simulink model "simulink_30_03"  (R2021a)
settings: Solver=FixedStepAuto  StartTime=0.0  StopTime=200  FixedStep=0.02  RelTol=1e-6
undefined symbols (not defined in the file): D_e, J_c, psi_sig, U_sig, V_sig
libraries: pid_lib x6, simulink x5, sharedutil x5, dspswit3 x1, aerolibutil x1
(part 1 of 3)
settings Model: Creator=frede  LastModifiedBy=frede
settings DataIOCC: SaveFormat=StructureWithTime  ReturnWorkspaceOutputs=off
settings OptimizationCC: BlockReduction=off  BufferReuse=off
settings DebuggingCC: AlgebraicLoopMsg=none  UnconnectedInputMsg=none  UnconnectedOutputMsg=none  UnconnectedLineMsg=none

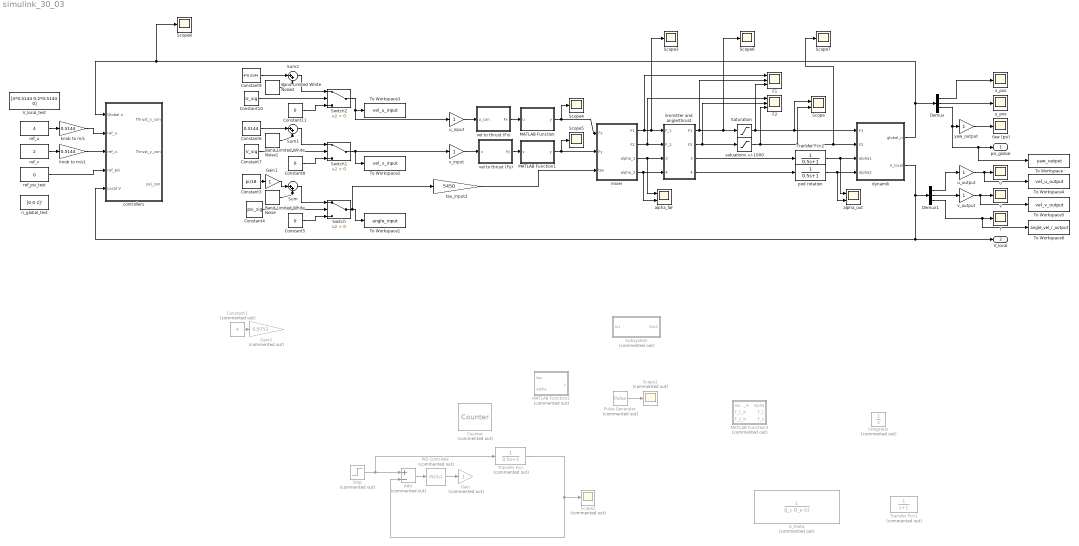
== system simulink_30_03 ==
  Add : Sum  Commented=on  Inputs=+-
  Band-Limited White Noise : simulink/Sources/Band-Limited White Noise  Cov=[0.01]  Ts=0.1  seed=[23341]
  Band-Limited White Noise1 : simulink/Sources/Band-Limited White Noise  Cov=[0.01]  Ts=0.1  seed=[23341]
  Band-Limited White Noise2 : simulink/Sources/Band-Limited White Noise  Cov=[0.01]  Ts=0.1  seed=[23341]
  Constant1 : Constant  Commented=on  Value=4
  Constant10 : Constant  Value=U_sig
  Constant11 : Constant  Value=0
  Constant3 : Constant  Value=pi/18
  Constant4 : Constant  Value=psi_sig
  Constant5 : Constant  Value=0
  Constant6 : Constant  Value=0.5144
  Constant7 : Constant  Value=V_sig
  Constant8 : Constant  Value=0
  Constant9 : Constant  Value=4*0.5144
  Counter : dspswit3/Counter  Commented=on  Direction=Up  CountEvent=Rising edge  CounterSize=User defined  MaxCount=500  InitialCount=0  Output=Count and Hit  HitValue=32  ResetInput=on  SamplesPerFrame=1  Ts=1  CntDtype=double  HitDtype=Logical
  Demux : Demux  Outputs=3
  Demux1 : Demux  Outputs=3
  F1 : Scope  NumInputPorts=3
  F2 : Scope  NumInputPorts=3
  G_theta : TransferFcn  Commented=on  Denominator=[J_c D_e 0]
  Gain : Gain  Commented=on
  Gain1 : Gain
  Gain3 : Gain  Commented=on  Gain=0.9752
  Integrator : Integrator  Commented=on
  MATLAB Function : MATLAB Function  TreatAsAtomicUnit=on
  MATLAB Function1 : MATLAB Function  TreatAsAtomicUnit=on
  MATLAB Function2 : MATLAB Function  Commented=on  TreatAsAtomicUnit=on
  MATLAB Function3 : MATLAB Function  Commented=on  TreatAsAtomicUnit=on
  PID Controller : pid_lib/PID Controller  Commented=on  Controller=PID  Form=Parallel  TimeDomain=Continuous-time  UseExternalTs=off  SampleTime=-1  IntegratorMethod=Forward Euler  FilterMethod=Forward Euler  ControllerParametersSource=internal  P=1.8562414179979  I=1.03694595494162  D=-0.170611805707441  UseFilter=on  N=7.0571761358123  TunerSelectOption=Transfer Function Based (PID Tuner App)  InitialConditionSource=internal  InitialConditionForIntegrator=0  InitialConditionForFilter=0  DifferentiatorICPrevScaledInput=0  ExternalReset=none  TrackingMode=off  Kt=1  LimitOutput=off  SatLimitsSource=internal  UpperSaturationLimit=inf  LowerSaturationLimit=-inf  LinearizeAsGain=on  AntiWindupMode=none  Kb=1  POutMin=[]  POutMax=[]  IOutMin=[]  IOutMax=[]  DOutMin=[]  DOutMax=[]  NOutMin=[]  NOutMax=[]  SumOutMin=[]  SumOutMax=[]  SaturationOutMin=[]  SaturationOutMax=[]  PParamMin=[]  PParamMax=[]  IParamMin=[]  IParamMax=[]  DParamMin=[]  DParamMax=[]  NParamMin=[]  NParamMax=[]  KbParamMin=[]  KbParamMax=[]  KtParamMin=[]  KtParamMax=[]  KbOutMin=[]  KbOutMax=[]  KtOutMin=[]  KtOutMax=[]  IntegratorOutMin=[]  IntegratorOutMax=[]  FilterOutMin=[]  FilterOutMax=[]  SumI1OutMin=[]  SumI1OutMax=[]  SumI2OutMin=[]  SumI2OutMax=[]  SumI3OutMin=[]  SumI3OutMax=[]  SumI4OutMin=[]  SumI4OutMax=[]  SumDOutMin=[]  SumDOutMax=[]  DifferentiatorOutMin=[]  DifferentiatorOutMax=[]  FilterDiffOutCoefMin=[]  FilterDiffOutCoefMax=[]  ReciprocalOutMin=[]  ReciprocalOutMax=[]  SumDenOutMin=[]  SumDenOutMax=[]  SumNumOutMin=[]  SumNumOutMax=[]  DivideOutMin=[]  DivideOutMax=[]  UdiffTsProdOutMin=[]  UdiffTsProdOutMax=[]  NTsProdOutMin=[]  NTsProdOutMax=[]  UintegralTsProdOutMin=[]  UintegralTsProdOutMax=[]  UngainTsProdOutMin=[]  UngainTsProdOutMax=[]  IntegratorContinuousStateAttributes=''  IntegratorStateMustResolveToSignalObject=off  IntegratorRTWStateStorageClass=Auto  FilterContinuousStateAttributes=''  FilterStateMustResolveToSignalObject=off  FilterRTWStateStorageClass=Auto  ParallelPVariant=InternalParameters  IdealPVariant=Disabled  IVariant=InternalParameters  DVariant=InternalParameters  IntegratorVariant=Continuous  SatVariant=Disabled  AWVariant=Passthrough  PCopyVariant=Disabled  TRVariant=Disabled  FdbkBlocksVariant=Forward  IdealPFdbkVariant=Disabled  SatFdbkVariant=Disabled  DerivativeFilterVariant=ContFilter  NVariant=InternalParameters  NCopyVariant=Disabled  FilterICVariant=InternalICsFilter  IntegratorICVariant=InternalICs  ExternalResetVariant=Disabled  TRSumVariant=Passthrough  SumFdbkVariant=Disabled  SumVariant=Sum_PID  TsampFilterVariant=InternalTs  TsampNgainVariant=Passthrough  TsampIntegralVariant=Passthrough  ExternalSaturationOutDataTypeStr=Inherit: Same as second input
  Pulse Generator : DiscretePulseGenerator  Commented=on  PulseType=Time based  Period=0.02222  PulseWidth=5
  Saturation : Saturate  UpperLimit=1000  LowerLimit=-1000
  Scope : Scope  NumInputPorts=2
  Scope1 : Scope  Commented=on
  Scope2 : Scope  Commented=on
  Scope{3..8} (6 alike) : Scope
  Step : Step  Commented=on  Time=0  After=0.78  SampleTime=0
  Subsystem : Subsystem  Commented=on
  Sum : Sum  Inputs=|++
  Sum1 : Sum  Inputs=|++
  Sum2 : Sum  Inputs=|++
  Switch : Switch  Criteria=u2 > Threshold
  Switch1 : Switch  Criteria=u2 > Threshold
  Switch2 : Switch  Criteria=u2 > Threshold
  To Workspace : ToWorkspace  VariableName=yaw_output  SaveFormat=Timeseries  SampleTime=-1
  To Workspace1 : ToWorkspace  VariableName=angle_input  SaveFormat=Timeseries  SampleTime=-1
  To Workspace2 : ToWorkspace  VariableName=vel_v_input  SaveFormat=Timeseries  SampleTime=-1
  To Workspace3 : ToWorkspace  VariableName=vel_u_input  SaveFormat=Timeseries  SampleTime=-1
  To Workspace4 : ToWorkspace  VariableName=vel_u_output  SaveFormat=Timeseries  SampleTime=-1
  To Workspace5 : ToWorkspace  VariableName=vel_v_output  SaveFormat=Timeseries  SampleTime=-1
  To Workspace6 : ToWorkspace  VariableName=angle_vel_r_output  SaveFormat=Timeseries  SampleTime=-1
  Transfer Fcn : TransferFcn  Commented=on  Denominator=[0.5 1]
  Transfer Fcn1 : TransferFcn  Commented=on  Denominator=[1 1]
  Transfer Fcn2 : TransferFcn  Denominator=[0.5 1]
  V_local_test : Constant  Value=[4*0.5144 0.2*0.5144 0]
  Yaw (psi) : Scope
  alpha_før : Scope  NumInputPorts=2
  alpha_out : Scope  NumInputPorts=2
  controllers : Subsystem
  dynamik : Subsystem
  knob to m/s : Gain  Gain=0.5144
  knob to m/s1 : Gain  Gain=0.5144
  "limmitter and angle/thrust " : MATLAB Function  TreatAsAtomicUnit=on
  mixer : Subsystem
  n_global_test : Constant  Value=[0 0 2]'
  pod rotation : TransferFcn  Denominator=[0.5 1]
  r : Scope
  ref_psi_test : Constant  Value=0
  ref_u : Constant  Value=4
  ref_v : Constant  Value=2
  "satuations +/-1000 " : Saturate  UpperLimit=1000  LowerLimit=-1000
  tau_input2 : Gain  Gain=5450
  u : Scope
  u_input : Gain
  u_output : Gain
  v : Scope
  v_input : Gain
  v_output : Gain
  vel to thrust (Fx) : MATLAB Function  TreatAsAtomicUnit=on
  vel to thrust (Fy) : MATLAB Function  TreatAsAtomicUnit=on
  x_pos : Scope
  y_pos : Scope
  yaw_output : Gain
  psi_global : Outport
  V_local : Outport  Port=2
  wires:
  yaw_output/1 -> Yaw (psi)/1
  Pulse Generator/1 -> Scope1/1
  ref_v/1 -> knob to m/s1/1
  v_output/1 -> To Workspace5/1, v/1
  tau_input2/1 -> mixer/3(tau)
  Demux/2 -> y_pos/1
  ref_u/1 -> knob to m/s/1
  vel to thrust (Fy)/1(Fy) -> MATLAB Function1/1(v)
  ref_psi_test/1 -> controllers/4(ref_psi.)
  Demux1/2 -> v_output/1
  knob to m/s/1 -> controllers/2(ref_u.)
  knob to m/s1/1 -> controllers/3(ref_v.)
  Demux1/1 -> u_output/1
  Sum/1 -> Switch/1
  Demux/1 -> x_pos/1
  dynamik/2(V_local) -> controllers/5(Local V), V_local/1, Demux1/1
  Demux/3 -> yaw_output/1, To Workspace/1, psi_global/1
  dynamik/1(global_n) -> Scope8/1, controllers/1(Global n), Demux/1
  vel to thrust (Fx)/1(Fx) -> MATLAB Function/1(u)
  Add/1 -> PID Controller/1
  Step/1 -> Transfer Fcn/1, Add/1
  Transfer Fcn/1 -> Scope2/1, Add/2
  PID Controller/1 -> Gain/1
  Transfer Fcn2/1 -> alpha_out/1, dynamik/3(alpha1)
  pod rotation/1 -> alpha_out/2, dynamik/4(alpha2)
  "satuations +/-1000 "/1 -> Scope/2, Scope7/1, dynamik/2(F2), F2/3
  "limmitter and angle/thrust "/1(F1) -> F1/2, Scope6/1, Saturation/1
  mixer/1(F1) -> F1/1, Scope3/1, "limmitter and angle/thrust "/1(F_1)
  mixer/2(F2) -> F2/1, "limmitter and angle/thrust "/2(F_2)
  "limmitter and angle/thrust "/2(F2) -> F2/2, "satuations +/-1000 "/1
  mixer/3(alpha_1) -> "limmitter and angle/thrust "/3(alpha_in_1), alpha_før/1
  "limmitter and angle/thrust "/4(alpha2) -> pod rotation/1
  "limmitter and angle/thrust "/3(alpha1) -> Transfer Fcn2/1
  MATLAB Function/1(y) -> Scope4/1, mixer/1(Fx)
  MATLAB Function1/1(y) -> Scope5/1, mixer/2(Fy)
  mixer/4(alpha_2) -> alpha_før/2, "limmitter and angle/thrust "/4(alpha_in_2)
  Saturation/1 -> Scope/1, dynamik/1(F1), F1/3
  Band-Limited White Noise/1 -> Sum/2
  Constant3/1 -> Gain1/1
  u_input/1 -> vel to thrust (Fx)/1(u_con)
  v_input/1 -> vel to thrust (Fy)/1(v)
  Gain1/1 -> Sum/1
  Constant4/1 -> Switch/2
  Constant5/1 -> Switch/3
  Constant6/1 -> Sum1/1
  Sum1/1 -> Switch1/1
  Constant7/1 -> Switch1/2
  Constant8/1 -> Switch1/3
  Band-Limited White Noise1/1 -> Sum1/2
  Constant10/1 -> Switch2/2
  Sum2/1 -> Switch2/1
  Constant11/1 -> Switch2/3
  Constant9/1 -> Sum2/1
  Band-Limited White Noise2/1 -> Sum2/2
  Demux1/3 -> To Workspace6/1, r/1
  Constant1/1 -> Gain3/1
  Switch2/1 -> u_input/1, To Workspace3/1
  Switch/1 -> tau_input2/1, To Workspace1/1
  u_output/1 -> To Workspace4/1, u/1
  Switch1/1 -> v_input/1, To Workspace2/1

== system simulink_30_03/Subsystem ==
  In1 : Inport
  MATLAB Function : MATLAB Function  TreatAsAtomicUnit=on
  Out1 : Outport
  wires:
  In1/1 -> Out1/1

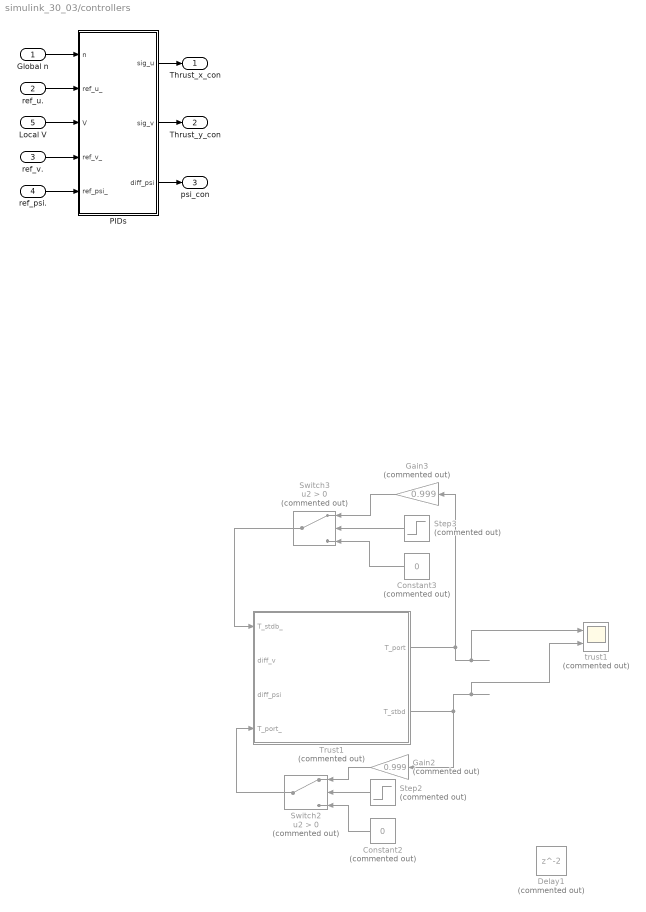
== system simulink_30_03/controllers ==
  Global n : Inport
  ref_u. : Inport  Port=2
  ref_v. : Inport  Port=3
  ref_psi. : Inport  Port=4
  Local V : Inport  Port=5
  Constant2 : Constant  Commented=on  Value=0
  Constant3 : Constant  Commented=on  Value=0
  Delay1 : Delay  Commented=on
  Gain2 : Gain  Commented=on  Gain=0.999
  Gain3 : Gain  Commented=on  Gain=0.999
  PIDs : Subsystem
  Step2 : Step  Commented=on  Time=0  SampleTime=0
  Step3 : Step  Commented=on  Time=0  SampleTime=0
  Switch2 : Switch  Commented=on  Criteria=u2 > Threshold
  Switch3 : Switch  Commented=on  Criteria=u2 > Threshold
  Trust1 : Subsystem  Commented=on
  trust1 : Scope  Commented=on  NumInputPorts=2
  Thrust_x_con : Outport
  Thrust_y_con : Outport  Port=2
  psi_con : Outport  Port=3
  wires:
  ref_u./1 -> PIDs/2(ref_u_)
  Global n/1 -> PIDs/1(n)
  Local V/1 -> PIDs/3(V)
  ref_v./1 -> PIDs/4(ref_v_)
  Switch3/1 -> Trust1/1(T_stdb_)
  Switch2/1 -> Trust1/4(T_port_)
  Gain2/1 -> Switch2/1
  Gain3/1 -> Switch3/1
  Step3/1 -> Switch3/2
  Constant3/1 -> Switch3/3
  Step2/1 -> Switch2/2
  Trust1/1(T_port) -> trust1/1, Gain3/1
  Trust1/2(T_stbd) -> trust1/2, Gain2/1
  Constant2/1 -> Switch2/3
  PIDs/3(diff_psi) -> psi_con/1
  PIDs/1(sig_u) -> Thrust_x_con/1
  PIDs/2(sig_v) -> Thrust_y_con/1
  ref_psi./1 -> PIDs/5(ref_psi_)

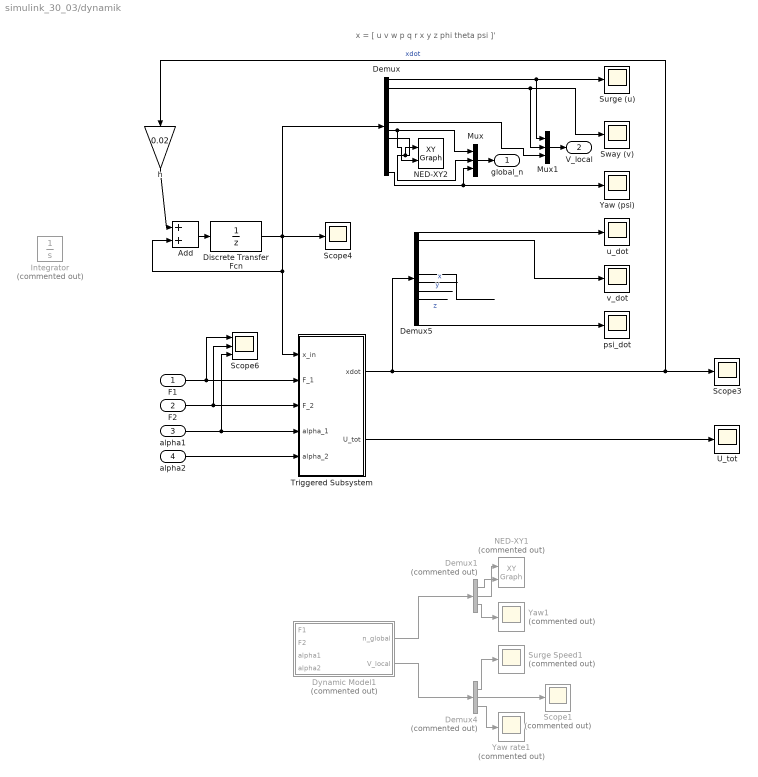
== system simulink_30_03/dynamik ==
  note: x = [ u v w p q r x y z phi theta psi ]'
  F1 : Inport
  F2 : Inport  Port=2
  alpha1 : Inport  Port=3
  alpha2 : Inport  Port=4
  Add : Sum
  Demux : Demux  Outputs=12
  Demux1 : Demux  Commented=on  Outputs=3
  Demux4 : Demux  Commented=on  Outputs=3
  Demux5 : Demux  Outputs=12
  Discrete Transfer Fcn : DiscreteTransferFcn  Denominator=[ 1 0]  SampleTime=0.02
  Dynamic Model1 : Subsystem  Commented=on
  Integrator : Integrator  Commented=on
  Mux : Mux  Inputs=3
  Mux1 : Mux  Inputs=3
  NED-XY1 : simulink/Sinks/XY Graph  Commented=on  xmin=-1000  xmax=1000  ymin=-1000  ymax=1000  st=-1
  NED-XY2 : simulink/Sinks/XY Graph  xmin=-1000  xmax=1000  ymin=-1000  ymax=1000  st=-1
  Scope1 : Scope  Commented=on
  Scope3 : Scope
  Scope4 : Scope
  Scope6 : Scope  NumInputPorts=3
  Surge (u) : Scope
  Surge Speed1 : Scope  Commented=on
  Sway (v) : Scope
  Triggered Subsystem : Subsystem  TreatAsAtomicUnit=on
  U_tot : Scope
  Yaw (psi) : Scope
  Yaw rate1 : Scope  Commented=on
  Yaw1 : Scope  Commented=on
  h : Gain  Gain=0.02
  psi_dot : Scope
  u_dot : Scope
  v_dot : Scope
  global_n : Outport
  V_local : Outport  Port=2
  wires:
  Demux1/3 -> Yaw1/1
  Demux4/3 -> Yaw rate1/1
  Demux1/2 -> NED-XY1/1
  Demux4/2 -> Scope1/1
  Demux1/1 -> NED-XY1/2
  Demux4/1 -> Surge Speed1/1
  Dynamic Model1/1(n_global) -> Demux1/1
  Dynamic Model1/2(V_local) -> Demux4/1
  F1/1 -> Scope6/1, Triggered Subsystem/2(F_1)
  F2/1 -> Scope6/2, Triggered Subsystem/3(F_2)
  alpha1/1 -> Scope6/3, Triggered Subsystem/4(alpha_1)
  alpha2/1 -> Triggered Subsystem/5(alpha_2)
  h/1 -> Add/1
  Add/1 -> Discrete Transfer Fcn/1
  Triggered Subsystem/1(xdot) -> Demux5/1, Scope3/1, h/1  "xdot"
  Triggered Subsystem/2(U_tot) -> U_tot/1
  Demux/8 -> Mux/2, NED-XY2/1
  Demux/7 -> NED-XY2/2, Mux/1
  Discrete Transfer Fcn/1 -> Scope4/1, Demux/1, Add/2, Triggered Subsystem/1(x_in)
  Demux/1 -> Surge (u)/1, Mux1/1
  Demux/12 -> Mux/3, Yaw (psi)/1
  Demux/2 -> Mux1/2, Sway (v)/1
  Mux/1 -> global_n/1
  Demux5/12 -> psi_dot/1
  Demux5/2 -> v_dot/1
  Demux5/1 -> u_dot/1
  Demux5/9 -> ?  "z"
  Demux5/7 -> ?  "x"
  Demux5/8 -> ?  "y"
  Mux1/1 -> V_local/1
  Demux5/6 -> ?
  Demux/6 -> Mux1/3

== system simulink_30_03/mixer ==
  Fx : Inport
  Fy : Inport  Port=2
  tau : Inport  Port=3
  MATLAB Function : MATLAB Function  TreatAsAtomicUnit=on
  d : Constant  Value=1.3395
  F1 : Outport
  F2 : Outport  Port=2
  alpha_1 : Outport  Port=3
  alpha_2 : Outport  Port=4
  wires:
  d/1 -> MATLAB Function/4(d)
  MATLAB Function/1(F_1) -> F1/1
  Fx/1 -> MATLAB Function/1(F_x)
  Fy/1 -> MATLAB Function/2(F_y)
  tau/1 -> MATLAB Function/3(tau)
  MATLAB Function/2(F_2) -> F2/1
  MATLAB Function/3(alpha1) -> alpha_1/1
  MATLAB Function/4(alpha2) -> alpha_2/1

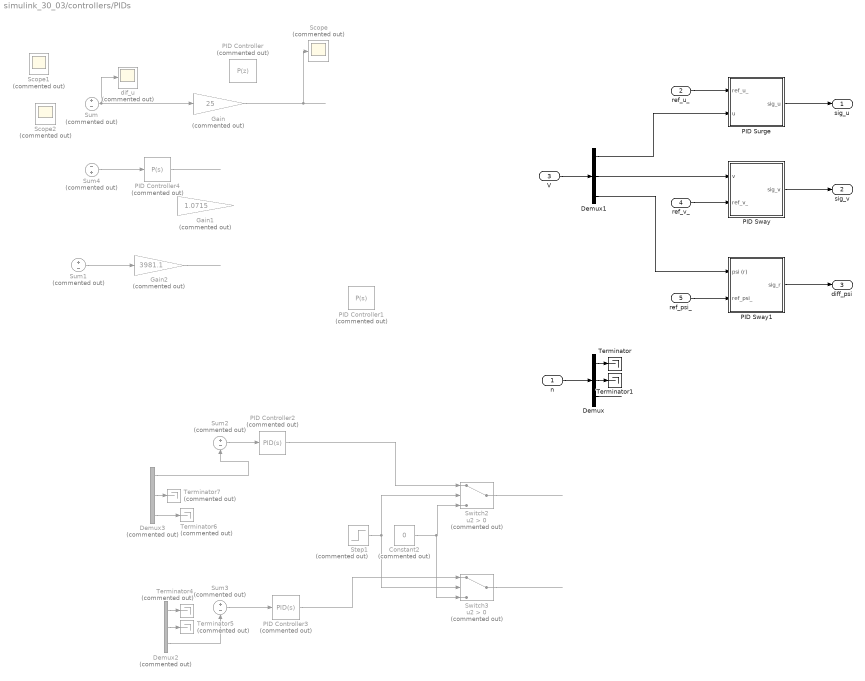
== system simulink_30_03/controllers/PIDs ==
  n : Inport
  ref_u_ : Inport  Port=2
  V : Inport  Port=3
  ref_v_ : Inport  Port=4
  ref_psi_ : Inport  Port=5
  Constant2 : Constant  Commented=on  Value=0
  Demux : Demux  Outputs=3
  Demux1 : Demux  Outputs=3
  Demux2 : Demux  Commented=on  Outputs=3
  Demux3 : Demux  Commented=on  Outputs=3
  Gain : Gain  Commented=on  Gain=25
  Gain1 : Gain  Commented=on  Gain=1.0715
  Gain2 : Gain  Commented=on  Gain=3981.1
  PID Controller : pid_lib/PID Controller  Commented=on  Controller=P  Form=Parallel  TimeDomain=Discrete-time  UseExternalTs=off  SampleTime=0.001  IntegratorMethod=Forward Euler  FilterMethod=Forward Euler  ControllerParametersSource=internal  P=0.9572  I=1  D=0  UseFilter=on  N=100  TunerSelectOption=Transfer Function Based (PID Tuner App)  InitialConditionSource=internal  InitialConditionForIntegrator=0  InitialConditionForFilter=0  DifferentiatorICPrevScaledInput=0  ExternalReset=none  TrackingMode=off  Kt=1  LimitOutput=off  SatLimitsSource=internal  UpperSaturationLimit=inf  LowerSaturationLimit=-inf  LinearizeAsGain=on  AntiWindupMode=none  Kb=1  POutMin=[]  POutMax=[]  IOutMin=[]  IOutMax=[]  DOutMin=[]  DOutMax=[]  NOutMin=[]  NOutMax=[]  SumOutMin=[]  SumOutMax=[]  SaturationOutMin=[]  SaturationOutMax=[]  PParamMin=[]  PParamMax=[]  IParamMin=[]  IParamMax=[]  DParamMin=[]  DParamMax=[]  NParamMin=[]  NParamMax=[]  KbParamMin=[]  KbParamMax=[]  KtParamMin=[]  KtParamMax=[]  KbOutMin=[]  KbOutMax=[]  KtOutMin=[]  KtOutMax=[]  IntegratorOutMin=[]  IntegratorOutMax=[]  FilterOutMin=[]  FilterOutMax=[]  SumI1OutMin=[]  SumI1OutMax=[]  SumI2OutMin=[]  SumI2OutMax=[]  SumI3OutMin=[]  SumI3OutMax=[]  SumI4OutMin=[]  SumI4OutMax=[]  SumDOutMin=[]  SumDOutMax=[]  DifferentiatorOutMin=[]  DifferentiatorOutMax=[]  FilterDiffOutCoefMin=[]  FilterDiffOutCoefMax=[]  ReciprocalOutMin=[]  ReciprocalOutMax=[]  SumDenOutMin=[]  SumDenOutMax=[]  SumNumOutMin=[]  SumNumOutMax=[]  DivideOutMin=[]  DivideOutMax=[]  UdiffTsProdOutMin=[]  UdiffTsProdOutMax=[]  NTsProdOutMin=[]  NTsProdOutMax=[]  UintegralTsProdOutMin=[]  UintegralTsProdOutMax=[]  UngainTsProdOutMin=[]  UngainTsProdOutMax=[]  IntegratorContinuousStateAttributes=''  IntegratorStateMustResolveToSignalObject=off  IntegratorRTWStateStorageClass=Auto  FilterContinuousStateAttributes=''  FilterStateMustResolveToSignalObject=off  FilterRTWStateStorageClass=Auto  ParallelPVariant=InternalParameters  IdealPVariant=Disabled  IVariant=InternalParameters  DVariant=InternalParameters  IntegratorVariant=Continuous  SatVariant=Disabled  AWVariant=Passthrough  PCopyVariant=Disabled  TRVariant=Disabled  FdbkBlocksVariant=Forward  IdealPFdbkVariant=Disabled  SatFdbkVariant=Disabled  DerivativeFilterVariant=ContFilter  NVariant=InternalParameters  NCopyVariant=Disabled  FilterICVariant=InternalICsFilter  IntegratorICVariant=InternalICs  ExternalResetVariant=Disabled  TRSumVariant=Passthrough  SumFdbkVariant=Disabled  SumVariant=Sum_PID  TsampFilterVariant=InternalTs  TsampNgainVariant=Passthrough  TsampIntegralVariant=Passthrough  ExternalSaturationOutDataTypeStr=Inherit: Same as second input
  PID Controller1 : pid_lib/PID Controller  Commented=on  Controller=P  Form=Parallel  TimeDomain=Continuous-time  UseExternalTs=off  SampleTime=-1  IntegratorMethod=Forward Euler  FilterMethod=Forward Euler  ControllerParametersSource=internal  P=3981.1  I=0.00289574585915178  D=6.03455227098632  UseFilter=on  N=202.272998620878  TunerSelectOption=Transfer Function Based (PID Tuner App)  InitialConditionSource=internal  InitialConditionForIntegrator=0  InitialConditionForFilter=0  DifferentiatorICPrevScaledInput=0  ExternalReset=none  TrackingMode=off  Kt=1  LimitOutput=off  SatLimitsSource=internal  UpperSaturationLimit=inf  LowerSaturationLimit=-inf  LinearizeAsGain=on  AntiWindupMode=none  Kb=1  POutMin=[]  POutMax=[]  IOutMin=[]  IOutMax=[]  DOutMin=[]  DOutMax=[]  NOutMin=[]  NOutMax=[]  SumOutMin=[]  SumOutMax=[]  SaturationOutMin=[]  SaturationOutMax=[]  PParamMin=[]  PParamMax=[]  IParamMin=[]  IParamMax=[]  DParamMin=[]  DParamMax=[]  NParamMin=[]  NParamMax=[]  KbParamMin=[]  KbParamMax=[]  KtParamMin=[]  KtParamMax=[]  KbOutMin=[]  KbOutMax=[]  KtOutMin=[]  KtOutMax=[]  IntegratorOutMin=[]  IntegratorOutMax=[]  FilterOutMin=[]  FilterOutMax=[]  SumI1OutMin=[]  SumI1OutMax=[]  SumI2OutMin=[]  SumI2OutMax=[]  SumI3OutMin=[]  SumI3OutMax=[]  SumI4OutMin=[]  SumI4OutMax=[]  SumDOutMin=[]  SumDOutMax=[]  DifferentiatorOutMin=[]  DifferentiatorOutMax=[]  FilterDiffOutCoefMin=[]  FilterDiffOutCoefMax=[]  ReciprocalOutMin=[]  ReciprocalOutMax=[]  SumDenOutMin=[]  SumDenOutMax=[]  SumNumOutMin=[]  SumNumOutMax=[]  DivideOutMin=[]  DivideOutMax=[]  UdiffTsProdOutMin=[]  UdiffTsProdOutMax=[]  NTsProdOutMin=[]  NTsProdOutMax=[]  UintegralTsProdOutMin=[]  UintegralTsProdOutMax=[]  UngainTsProdOutMin=[]  UngainTsProdOutMax=[]  IntegratorContinuousStateAttributes=''  IntegratorStateMustResolveToSignalObject=off  IntegratorRTWStateStorageClass=Auto  FilterContinuousStateAttributes=''  FilterStateMustResolveToSignalObject=off  FilterRTWStateStorageClass=Auto  ParallelPVariant=InternalParameters  IdealPVariant=Disabled  IVariant=InternalParameters  DVariant=InternalParameters  IntegratorVariant=Continuous  SatVariant=Disabled  AWVariant=Passthrough  PCopyVariant=Disabled  TRVariant=Disabled  FdbkBlocksVariant=Forward  IdealPFdbkVariant=Disabled  SatFdbkVariant=Disabled  DerivativeFilterVariant=ContFilter  NVariant=InternalParameters  NCopyVariant=Disabled  FilterICVariant=InternalICsFilter  IntegratorICVariant=InternalICs  ExternalResetVariant=Disabled  TRSumVariant=Passthrough  SumFdbkVariant=Disabled  SumVariant=Sum_PID  TsampFilterVariant=InternalTs  TsampNgainVariant=Passthrough  TsampIntegralVariant=Passthrough  ExternalSaturationOutDataTypeStr=Inherit: Same as second input
  PID Controller2 : pid_lib/PID Controller  Commented=on  Controller=PID  Form=Parallel  TimeDomain=Continuous-time  UseExternalTs=off  SampleTime=-1  IntegratorMethod=Forward Euler  FilterMethod=Forward Euler  ControllerParametersSource=internal  P=6.45174968659804  I=0  D=0  UseFilter=on  N=100  TunerSelectOption=Transfer Function Based (PID Tuner App)  InitialConditionSource=internal  InitialConditionForIntegrator=0  InitialConditionForFilter=0  DifferentiatorICPrevScaledInput=0  ExternalReset=none  TrackingMode=off  Kt=1  LimitOutput=off  SatLimitsSource=internal  UpperSaturationLimit=inf  LowerSaturationLimit=-inf  LinearizeAsGain=on  AntiWindupMode=none  Kb=1  POutMin=[]  POutMax=[]  IOutMin=[]  IOutMax=[]  DOutMin=[]  DOutMax=[]  NOutMin=[]  NOutMax=[]  SumOutMin=[]  SumOutMax=[]  SaturationOutMin=[]  SaturationOutMax=[]  PParamMin=[]  PParamMax=[]  IParamMin=[]  IParamMax=[]  DParamMin=[]  DParamMax=[]  NParamMin=[]  NParamMax=[]  KbParamMin=[]  KbParamMax=[]  KtParamMin=[]  KtParamMax=[]  KbOutMin=[]  KbOutMax=[]  KtOutMin=[]  KtOutMax=[]  IntegratorOutMin=[]  IntegratorOutMax=[]  FilterOutMin=[]  FilterOutMax=[]  SumI1OutMin=[]  SumI1OutMax=[]  SumI2OutMin=[]  SumI2OutMax=[]  SumI3OutMin=[]  SumI3OutMax=[]  SumI4OutMin=[]  SumI4OutMax=[]  SumDOutMin=[]  SumDOutMax=[]  DifferentiatorOutMin=[]  DifferentiatorOutMax=[]  FilterDiffOutCoefMin=[]  FilterDiffOutCoefMax=[]  ReciprocalOutMin=[]  ReciprocalOutMax=[]  SumDenOutMin=[]  SumDenOutMax=[]  SumNumOutMin=[]  SumNumOutMax=[]  DivideOutMin=[]  DivideOutMax=[]  UdiffTsProdOutMin=[]  UdiffTsProdOutMax=[]  NTsProdOutMin=[]  NTsProdOutMax=[]  UintegralTsProdOutMin=[]  UintegralTsProdOutMax=[]  UngainTsProdOutMin=[]  UngainTsProdOutMax=[]  IntegratorContinuousStateAttributes=''  IntegratorStateMustResolveToSignalObject=off  IntegratorRTWStateStorageClass=Auto  FilterContinuousStateAttributes=''  FilterStateMustResolveToSignalObject=off  FilterRTWStateStorageClass=Auto  ParallelPVariant=InternalParameters  IdealPVariant=Disabled  IVariant=InternalParameters  DVariant=InternalParameters  IntegratorVariant=Continuous  SatVariant=Disabled  AWVariant=Passthrough  PCopyVariant=Disabled  TRVariant=Disabled  FdbkBlocksVariant=Forward  IdealPFdbkVariant=Disabled  SatFdbkVariant=Disabled  DerivativeFilterVariant=ContFilter  NVariant=InternalParameters  NCopyVariant=Disabled  FilterICVariant=InternalICsFilter  IntegratorICVariant=InternalICs  ExternalResetVariant=Disabled  TRSumVariant=Passthrough  SumFdbkVariant=Disabled  SumVariant=Sum_PID  TsampFilterVariant=InternalTs  TsampNgainVariant=Passthrough  TsampIntegralVariant=Passthrough  ExternalSaturationOutDataTypeStr=Inherit: Same as second input
  PID Controller3 : pid_lib/PID Controller  Commented=on  Controller=PID  Form=Parallel  TimeDomain=Continuous-time  UseExternalTs=off  SampleTime=-1  IntegratorMethod=Forward Euler  FilterMethod=Forward Euler  ControllerParametersSource=internal  P=131.029347680275  I=1.01635655292668  D=2972.43198696455  UseFilter=on  N=131.214207944012  TunerSelectOption=Transfer Function Based (PID Tuner App)  InitialConditionSource=internal  InitialConditionForIntegrator=0  InitialConditionForFilter=0  DifferentiatorICPrevScaledInput=0  ExternalReset=none  TrackingMode=off  Kt=1  LimitOutput=off  SatLimitsSource=internal  UpperSaturationLimit=inf  LowerSaturationLimit=-inf  LinearizeAsGain=on  AntiWindupMode=none  Kb=1  POutMin=[]  POutMax=[]  IOutMin=[]  IOutMax=[]  DOutMin=[]  DOutMax=[]  NOutMin=[]  NOutMax=[]  SumOutMin=[]  SumOutMax=[]  SaturationOutMin=[]  SaturationOutMax=[]  PParamMin=[]  PParamMax=[]  IParamMin=[]  IParamMax=[]  DParamMin=[]  DParamMax=[]  NParamMin=[]  NParamMax=[]  KbParamMin=[]  KbParamMax=[]  KtParamMin=[]  KtParamMax=[]  KbOutMin=[]  KbOutMax=[]  KtOutMin=[]  KtOutMax=[]  IntegratorOutMin=[]  IntegratorOutMax=[]  FilterOutMin=[]  FilterOutMax=[]  SumI1OutMin=[]  SumI1OutMax=[]  SumI2OutMin=[]  SumI2OutMax=[]  SumI3OutMin=[]  SumI3OutMax=[]  SumI4OutMin=[]  SumI4OutMax=[]  SumDOutMin=[]  SumDOutMax=[]  DifferentiatorOutMin=[]  DifferentiatorOutMax=[]  FilterDiffOutCoefMin=[]  FilterDiffOutCoefMax=[]  ReciprocalOutMin=[]  ReciprocalOutMax=[]  SumDenOutMin=[]  SumDenOutMax=[]  SumNumOutMin=[]  SumNumOutMax=[]  DivideOutMin=[]  DivideOutMax=[]  UdiffTsProdOutMin=[]  UdiffTsProdOutMax=[]  NTsProdOutMin=[]  NTsProdOutMax=[]  UintegralTsProdOutMin=[]  UintegralTsProdOutMax=[]  UngainTsProdOutMin=[]  UngainTsProdOutMax=[]  IntegratorContinuousStateAttributes=''  IntegratorStateMustResolveToSignalObject=off  IntegratorRTWStateStorageClass=Auto  FilterContinuousStateAttributes=''  FilterStateMustResolveToSignalObject=off  FilterRTWStateStorageClass=Auto  ParallelPVariant=InternalParameters  IdealPVariant=Disabled  IVariant=InternalParameters  DVariant=InternalParameters  IntegratorVariant=Continuous  SatVariant=Disabled  AWVariant=Passthrough  PCopyVariant=Disabled  TRVariant=Disabled  FdbkBlocksVariant=Forward  IdealPFdbkVariant=Disabled  SatFdbkVariant=Disabled  DerivativeFilterVariant=ContFilter  NVariant=InternalParameters  NCopyVariant=Disabled  FilterICVariant=InternalICsFilter  IntegratorICVariant=InternalICs  ExternalResetVariant=Disabled  TRSumVariant=Passthrough  SumFdbkVariant=Disabled  SumVariant=Sum_PID  TsampFilterVariant=InternalTs  TsampNgainVariant=Passthrough  TsampIntegralVariant=Passthrough  ExternalSaturationOutDataTypeStr=Inherit: Same as second input
  PID Controller4 : pid_lib/PID Controller  Commented=on  Controller=P  Form=Parallel  TimeDomain=Continuous-time  UseExternalTs=off  SampleTime=-1  IntegratorMethod=Forward Euler  FilterMethod=Forward Euler  ControllerParametersSource=internal  P=1.0715  I=0.1  D=0.00005  UseFilter=on  N=684.920595200174  TunerSelectOption=Transfer Function Based (PID Tuner App)  InitialConditionSource=internal  InitialConditionForIntegrator=0  InitialConditionForFilter=0  DifferentiatorICPrevScaledInput=0  ExternalReset=none  TrackingMode=off  Kt=1  LimitOutput=off  SatLimitsSource=internal  UpperSaturationLimit=inf  LowerSaturationLimit=-inf  LinearizeAsGain=on  AntiWindupMode=none  Kb=1  POutMin=[]  POutMax=[]  IOutMin=[]  IOutMax=[]  DOutMin=[]  DOutMax=[]  NOutMin=[]  NOutMax=[]  SumOutMin=[]  SumOutMax=[]  SaturationOutMin=[]  SaturationOutMax=[]  PParamMin=[]  PParamMax=[]  IParamMin=[]  IParamMax=[]  DParamMin=[]  DParamMax=[]  NParamMin=[]  NParamMax=[]  KbParamMin=[]  KbParamMax=[]  KtParamMin=[]  KtParamMax=[]  KbOutMin=[]  KbOutMax=[]  KtOutMin=[]  KtOutMax=[]  IntegratorOutMin=[]  IntegratorOutMax=[]  FilterOutMin=[]  FilterOutMax=[]  SumI1OutMin=[]  SumI1OutMax=[]  SumI2OutMin=[]  SumI2OutMax=[]  SumI3OutMin=[]  SumI3OutMax=[]  SumI4OutMin=[]  SumI4OutMax=[]  SumDOutMin=[]  SumDOutMax=[]  DifferentiatorOutMin=[]  DifferentiatorOutMax=[]  FilterDiffOutCoefMin=[]  FilterDiffOutCoefMax=[]  ReciprocalOutMin=[]  ReciprocalOutMax=[]  SumDenOutMin=[]  SumDenOutMax=[]  SumNumOutMin=[]  SumNumOutMax=[]  DivideOutMin=[]  DivideOutMax=[]  UdiffTsProdOutMin=[]  UdiffTsProdOutMax=[]  NTsProdOutMin=[]  NTsProdOutMax=[]  UintegralTsProdOutMin=[]  UintegralTsProdOutMax=[]  UngainTsProdOutMin=[]  UngainTsProdOutMax=[]  IntegratorContinuousStateAttributes=''  IntegratorStateMustResolveToSignalObject=off  IntegratorRTWStateStorageClass=Auto  FilterContinuousStateAttributes=''  FilterStateMustResolveToSignalObject=off  FilterRTWStateStorageClass=Auto  ParallelPVariant=InternalParameters  IdealPVariant=Disabled  IVariant=InternalParameters  DVariant=InternalParameters  IntegratorVariant=Continuous  SatVariant=Disabled  AWVariant=Passthrough  PCopyVariant=Disabled  TRVariant=Disabled  FdbkBlocksVariant=Forward  IdealPFdbkVariant=Disabled  SatFdbkVariant=Disabled  DerivativeFilterVariant=ContFilter  NVariant=InternalParameters  NCopyVariant=Disabled  FilterICVariant=InternalICsFilter  IntegratorICVariant=InternalICs  ExternalResetVariant=Disabled  TRSumVariant=Passthrough  SumFdbkVariant=Disabled  SumVariant=Sum_PID  TsampFilterVariant=InternalTs  TsampNgainVariant=Passthrough  TsampIntegralVariant=Passthrough  ExternalSaturationOutDataTypeStr=Inherit: Same as second input
  PID Surge : Subsystem
  PID Sway : Subsystem
  PID Sway1 : Subsystem
  Scope : Scope  Commented=on
  Scope1 : Scope  Commented=on
  Scope2 : Scope  Commented=on
  Step1 : Step  Commented=on  Time=0  SampleTime=0
  Sum{,1..3} (4 alike) : Sum  Commented=on  Inputs=+|-
  Sum4 : Sum  Commented=on  Inputs=-|+
  Switch2 : Switch  Commented=on  Criteria=u2 > Threshold
  Switch3 : Switch  Commented=on  Criteria=u2 > Threshold
  Terminator : Terminator
  Terminator1 : Terminator
  Terminator{4..7} (4 alike) : Terminator  Commented=on
  dif_u : Scope  Commented=on
  sig_u : Outport
  sig_v : Outport  Port=2
  diff_psi : Outport  Port=3
  wires:
  Sum1/1 -> Gain2/1
  ? -> Scope1/1, Sum/1
  Constant2/1 -> Switch3/3, Switch2/3
  Demux2/1 -> Terminator4/1
  Demux3/2 -> Terminator7/1
  Switch3/1 -> ?
  Sum3/1 -> PID Controller3/1
  Sum2/1 -> PID Controller2/1
  Demux3/1 -> Sum2/2
  PID Controller3/1 -> Switch3/1
  Demux2/2 -> Terminator5/1
  Switch2/1 -> ?
  Demux3/3 -> Terminator6/1
  PID Controller2/1 -> Switch2/1
  Step1/1 -> Switch3/2, Switch2/2
  Demux2/3 -> Sum3/2
  PID Controller4/1 -> ?
  Sum4/1 -> PID Controller4/1
  ? -> Sum4/2
  Gain2/1 -> ?
  n/1 -> Demux/1
  Demux/3 -> ?
  Demux/1 -> Terminator/1
  Demux/2 -> Terminator1/1
  ? -> Sum1/2
  Gain/1 -> Scope/1
  Sum/1 -> Gain/1, dif_u/1
  Demux1/3 -> PID Sway1/1(psi (r))
  V/1 -> Demux1/1
  ref_u_/1 -> PID Surge/1(ref_u_)
  Demux1/1 -> PID Surge/2(u)
  PID Surge/1(sig_u) -> sig_u/1
  Demux1/2 -> PID Sway/1(v)
  ref_v_/1 -> PID Sway/2(ref_v_)
  PID Sway/1(sig_v) -> sig_v/1
  ref_psi_/1 -> PID Sway1/2(ref_psi_)
  PID Sway1/1(sig_r) -> diff_psi/1

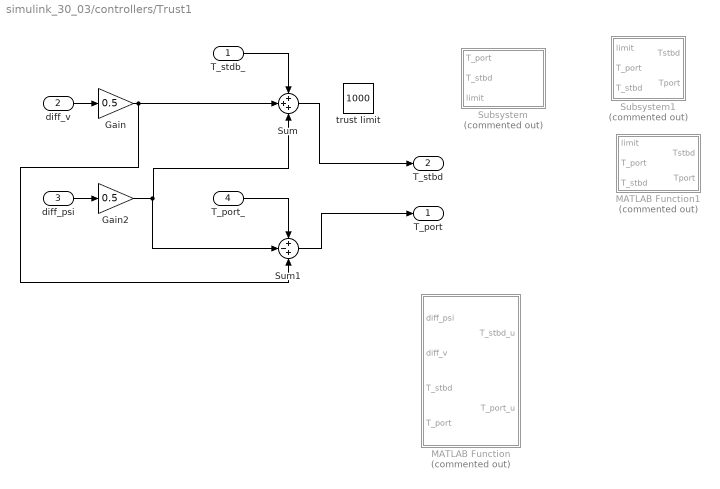
== system simulink_30_03/controllers/Trust1 ==
  T_stdb_ : Inport
  diff_v : Inport  Port=2
  diff_psi : Inport  Port=3
  T_port_ : Inport  Port=4
  Gain : Gain  Gain=0.5
  Gain2 : Gain  Gain=0.5
  MATLAB Function : MATLAB Function  Commented=on  TreatAsAtomicUnit=on
  MATLAB Function1 : MATLAB Function  Commented=on  TreatAsAtomicUnit=on
  Subsystem : Subsystem  Commented=on
  Subsystem1 : Subsystem  Commented=on
  Sum : Sum  Inputs=+++
  Sum1 : Sum  Inputs=+-+
  trust limit : Constant  Value=1000
  T_port : Outport
  T_stbd : Outport  Port=2
  wires:
  diff_v/1 -> Gain/1
  T_stdb_/1 -> Sum/1
  T_port_/1 -> Sum1/1
  Gain/1 -> Sum1/3, Sum/2
  diff_psi/1 -> Gain2/1
  Gain2/1 -> Sum/3, Sum1/2
  Sum/1 -> T_stbd/1
  Sum1/1 -> T_port/1

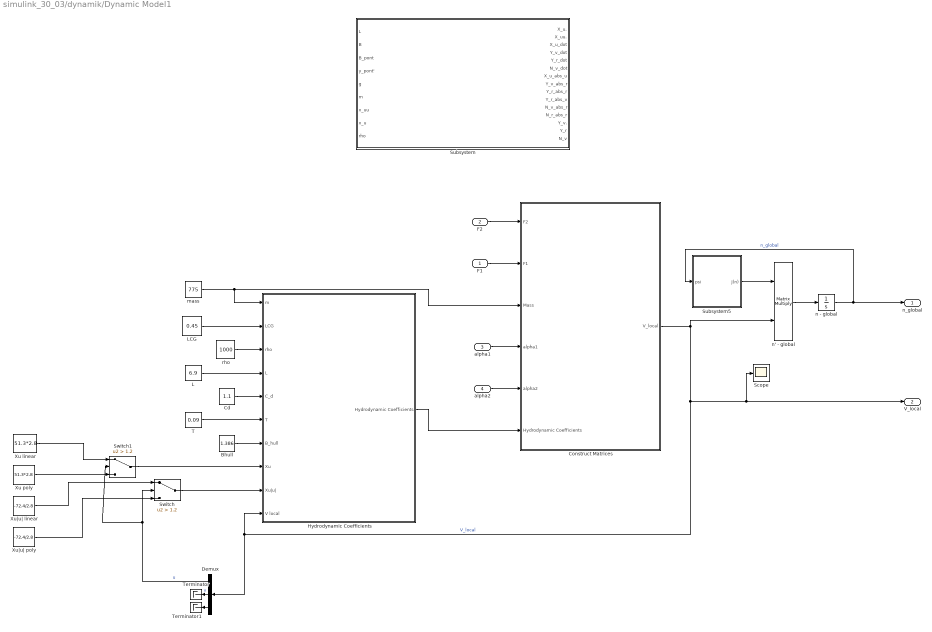
== system simulink_30_03/dynamik/Dynamic Model1 ==
  F1 : Inport
  F2 : Inport  Port=2
  alpha1 : Inport  Port=3
  alpha2 : Inport  Port=4
  "Bhull " : Constant  Value=1.386
  Cd : Constant  Value=1.1
  Construct Matrices : Subsystem
  Demux : Demux  Outputs=3
  Hydrodynamic Coefficients : Subsystem
  L : Constant  Value=6.9
  LCG : Constant  Value=0.45
  Scope : Scope
  Subsystem : Subsystem
  Subsystem5 : Subsystem
  Switch : Switch  Criteria=u2 > Threshold  Threshold=1.2
  Switch1 : Switch  Criteria=u2 > Threshold  Threshold=1.2
  T : Constant  Value=0.09
  Terminator : Terminator
  Terminator1 : Terminator
  Xu linear : Constant  Value=51.3*2.8
  Xu poly : Constant  Value=51.3*2.8
  Xu|u| linear : Constant  Value=-72.4/2.8
  Xu|u| poly : Constant  Value=-72.4/2.8
  mass : Constant  Value=775
  n - global : Integrator  InitialCondition=[0 0 0]
  n' - global : Product  Multiplication=Matrix(*)
  rho : Constant  Value=1000
  n_global : Outport  VectorParamsAs1DForOutWhenUnconnected=off
  V_local : Outport  Port=2  VectorParamsAs1DForOutWhenUnconnected=off
  wires:
  n - global/1 -> Subsystem5/1(psi), n_global/1  "n_global"
  Cd/1 -> Hydrodynamic Coefficients/5(C_d)
  Construct Matrices/1(V_local) -> n' - global/2, Demux/1, Hydrodynamic Coefficients/10(V local), Scope/1, V_local/1  "V_local"
  n' - global/1 -> n - global/1
  Subsystem5/1(J(n)) -> n' - global/1
  rho/1 -> Hydrodynamic Coefficients/3(rho)
  L/1 -> Hydrodynamic Coefficients/4(L)
  F2/1 -> Construct Matrices/1(F2)
  F1/1 -> Construct Matrices/2(F1)
  mass/1 -> Hydrodynamic Coefficients/1(m), Construct Matrices/3("Mass ")
  Hydrodynamic Coefficients/1("Hydrodynamic Coefficients ") -> Construct Matrices/6(Hydrodynamic Coefficients)
  T/1 -> Hydrodynamic Coefficients/6(T)
  "Bhull "/1 -> Hydrodynamic Coefficients/7(B_hull)
  Switch/1 -> Hydrodynamic Coefficients/9(Xu|u|)
  LCG/1 -> Hydrodynamic Coefficients/2(LCG)
  Demux/1 -> Switch1/2, Switch/2  "u"
  Xu|u| poly/1 -> Switch/3
  Xu|u| linear/1 -> Switch/1
  Switch1/1 -> Hydrodynamic Coefficients/8(Xu)
  Xu poly/1 -> Switch1/3
  Xu linear/1 -> Switch1/1
  Demux/3 -> Terminator1/1
  Demux/2 -> Terminator/1  "v"
  alpha1/1 -> Construct Matrices/4(alpha1)
  alpha2/1 -> Construct Matrices/5(alpha2)

== system simulink_30_03/dynamik/Triggered Subsystem ==
  note: x = [ u v w p q r x y z phi theta psi ]'
  x_in : Inport
  F_1 : Inport  Port=2
  F_2 : Inport  Port=3
  alpha_1 : Inport  Port=4
  alpha_2 : Inport  Port=5
  Demux : Demux  Outputs=12
  MATLAB Function : MATLAB Function  Commented=on  TreatAsAtomicUnit=on
  MATLAB Function1 : MATLAB Function  TreatAsAtomicUnit=on
  current vel : Constant  Value=0
  diretion of current : Constant  Value=0
  location of payload : Constant  Value=[0 0 -0.1]'
  n rpm : Constant  Value=[0 0]'
  payload : Constant  Value=0
  xdot : Outport
  U_tot : Outport  Port=2
  wires:
  F_1/1 -> MATLAB Function1/18(F_1)
  F_2/1 -> MATLAB Function1/19(F_2)
  alpha_1/1 -> MATLAB Function1/20(alpha_1)
  alpha_2/1 -> MATLAB Function1/21(alpha_2)
  location of payload/1 -> MATLAB Function1/15(rp)
  payload/1 -> MATLAB Function1/14(mp)
  current vel/1 -> MATLAB Function1/16(V_c)
  diretion of current/1 -> MATLAB Function1/17(beta_c)
  n rpm/1 -> MATLAB Function1/13(n)
  x_in/1 -> Demux/1
  MATLAB Function1/2(U_tot) -> U_tot/1
  MATLAB Function1/1(xdot) -> xdot/1
  Demux/1 -> MATLAB Function1/1(u)
  Demux/2 -> MATLAB Function1/2(v)
  Demux/3 -> MATLAB Function1/3(w)
  Demux/4 -> MATLAB Function1/4(p)
  Demux/5 -> MATLAB Function1/5(q)
  Demux/6 -> MATLAB Function1/6(r)
  Demux/7 -> MATLAB Function1/7(x)
  Demux/8 -> MATLAB Function1/8(y)
  Demux/9 -> MATLAB Function1/9(z)
  Demux/10 -> MATLAB Function1/10(phi)
  Demux/11 -> MATLAB Function1/11(theta)
  Demux/12 -> MATLAB Function1/12(psi)

== system simulink_30_03/controllers/PIDs/PID Surge ==
  ref_u_ : Inport
  u : Inport  Port=2
  Derivative : Derivative  Commented=through
  Integrator Limited : Integrator  LimitOutput=on  UpperSaturationLimit=3  LowerSaturationLimit=-3
  Kp : Gain  Gain=3
  Sum5 : Sum
  Sum6 : Sum  Inputs=|+-
  tau_d : Gain  Commented=through
  tau_i : Gain  Gain=1.3599
  sig_u : Outport
  wires:
  ref_u_/1 -> Sum6/1
  tau_i/1 -> Integrator Limited/1
  Sum5/1 -> sig_u/1
  Sum6/1 -> tau_i/1, Kp/1
  tau_d/1 -> Sum6/2
  Derivative/1 -> tau_d/1
  Kp/1 -> Sum5/2
  u/1 -> Derivative/1
  Integrator Limited/1 -> Sum5/1

== system simulink_30_03/controllers/PIDs/PID Sway ==
  v : Inport
  ref_v_ : Inport  Port=2
  Derivative1 : Derivative  Commented=through
  Integrator1 : Integrator
  Kp : Gain  Gain=2.15
  Sum7 : Sum
  Sum8 : Sum  Inputs=|+-
  tau_d1 : Gain  Commented=through
  tau_i : Gain  Gain=0
  sig_v : Outport
  wires:
  Sum8/1 -> Kp/1, Integrator1/1
  Integrator1/1 -> tau_i/1
  Kp/1 -> Sum7/2
  ref_v_/1 -> Sum8/1
  tau_i/1 -> Sum7/1
  Derivative1/1 -> tau_d1/1
  Sum7/1 -> sig_v/1
  tau_d1/1 -> Sum8/2
  v/1 -> Derivative1/1

== system simulink_30_03/controllers/PIDs/PID Sway1 ==
  psi (r) : Inport
  ref_psi_ : Inport  Port=2
  Derivative1 : Derivative
  Integrator1 : Integrator
  Kp : Gain
  Sum7 : Sum
  Sum8 : Sum  Inputs=|+-
  tau_d : Gain
  tau_i : Gain
  sig_r : Outport
  wires:
  Sum8/1 -> Kp/1, Integrator1/1
  Integrator1/1 -> tau_i/1
  Kp/1 -> Sum7/2
  ref_psi_/1 -> Sum8/1
  tau_i/1 -> Sum7/1
  Derivative1/1 -> tau_d/1
  Sum7/1 -> sig_r/1
  tau_d/1 -> Sum8/2
  psi (r)/1 -> Derivative1/1

== system simulink_30_03/controllers/Trust1/Subsystem ==
  "T_port " : Inport
  "T_stbd " : Inport  Port=2
  limit : Inport  Port=3

== system simulink_30_03/controllers/Trust1/Subsystem1 ==
  limit : Inport
  T_port : Inport  Port=2
  T_stbd : Inport  Port=3
  limit maks : MATLAB Function  TreatAsAtomicUnit=on
  limit min : MATLAB Function  TreatAsAtomicUnit=on
  Tstbd : Outport
  Tport : Outport  Port=2
  wires:
  limit/1 -> limit maks/1(limit), limit min/1(limit)
  T_stbd/1 -> limit min/3(T_stbd)
  T_port/1 -> limit min/2(T_port)
  limit min/2(Tport) -> limit maks/2(T_port)
  limit min/1(Tstbd) -> limit maks/3(T_stbd)
  limit maks/1(Tstbd) -> Tstbd/1
  limit maks/2(Tport) -> Tport/1

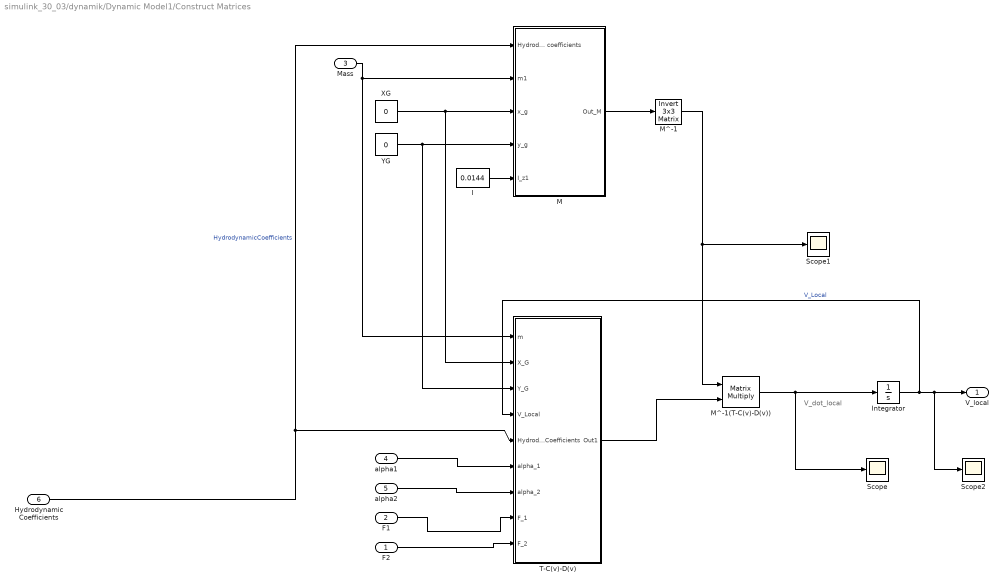
== system simulink_30_03/dynamik/Dynamic Model1/Construct Matrices ==
  note: V_dot_local
  F2 : Inport
  F1 : Inport  Port=2
  "Mass " : Inport  Port=3
  alpha1 : Inport  Port=4
  alpha2 : Inport  Port=5
  Hydrodynamic Coefficients : Inport  Port=6
  I : Constant  Value=0.0144
  Integrator : Integrator  InitialCondition=[0 0 0]
  M : Subsystem
  M^-1 : aerolibutil/Invert  3x3 Matrix
  M^-1(T-C(v)-D(v)) : Product  Multiplication=Matrix(*)
  Scope : Scope
  Scope1 : Scope
  Scope2 : Scope
  T-C(v)-D(v) : Subsystem
  XG : Constant  Value=0
  YG : Constant  Value=0
  V_local : Outport  VectorParamsAs1DForOutWhenUnconnected=off
  wires:
  Integrator/1 -> Scope2/1, V_local/1, T-C(v)-D(v)/4(V_Local)  "V_Local"
  M^-1(T-C(v)-D(v))/1 -> Scope/1, Integrator/1
  M/1(Out_M) -> M^-1/1
  Hydrodynamic Coefficients/1 -> M/1(Hydrodynamic coefficients), T-C(v)-D(v)/5(HydrodynamicCoefficients)  "HydrodynamicCoefficients"
  YG/1 -> M/4(y_g), T-C(v)-D(v)/3(Y_G)
  "Mass "/1 -> T-C(v)-D(v)/1(m), M/2(m1)
  XG/1 -> M/3(x_g), T-C(v)-D(v)/2(X_G)
  F1/1 -> T-C(v)-D(v)/8(F_1)
  F2/1 -> T-C(v)-D(v)/9(F_2)
  T-C(v)-D(v)/1(Out1) -> M^-1(T-C(v)-D(v))/2
  I/1 -> M/5(I_z1)
  alpha1/1 -> T-C(v)-D(v)/6(alpha_1)
  alpha2/1 -> T-C(v)-D(v)/7(alpha_2)
  M^-1/1 -> Scope1/1, M^-1(T-C(v)-D(v))/1

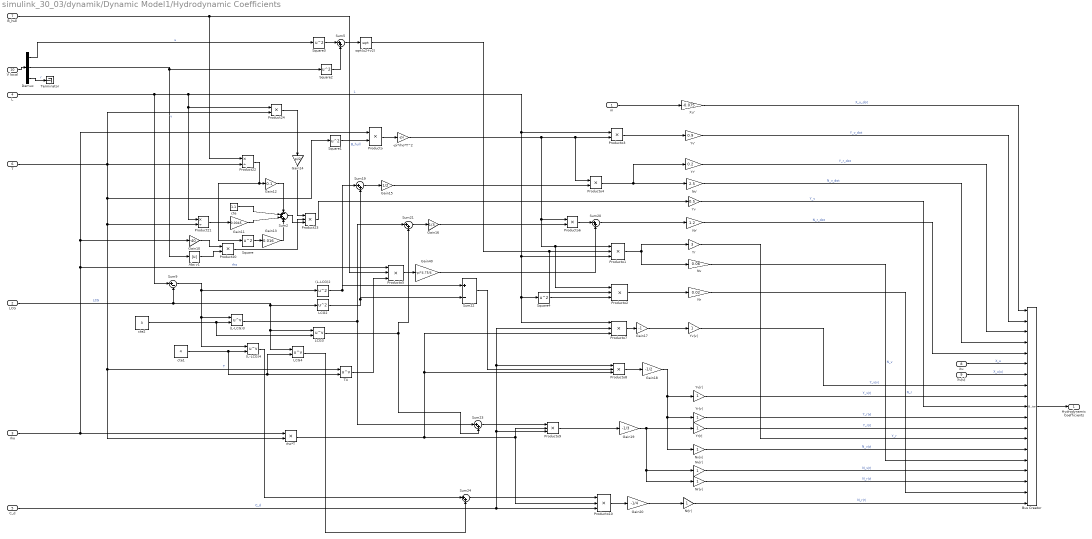
== system simulink_30_03/dynamik/Dynamic Model1/Hydrodynamic Coefficients ==
  m : Inport
  LCG : Inport  Port=2
  rho : Inport  Port=3
  L : Inport  Port=4
  C_d : Inport  Port=5
  T : Inport  Port=6
  B_hull : Inport  Port=7
  Xu : Inport  Port=8
  Xu|u| : Inport  Port=9
  V local : Inport  Port=10
  (L-LCG)2 : Math  Operator=square  SignedPower=on  SaturateOnIntegerOverflow=on
  (L-LCG)3 : Math  Operator=pow  SignedPower=on  SaturateOnIntegerOverflow=on
  (L-LCG)4 : Math  Operator=pow  SignedPower=on  SaturateOnIntegerOverflow=on
  -pi*rho*T^2 : Gain  Gain=-pi
  Abs v1 : Abs
  Bus Creator : BusCreator  Inputs=19
  Demux : Demux  Outputs=3
  Gain10 : Gain  Gain=-40
  Gain11 : Gain  Gain=0.0045
  Gain12 : Gain  Gain=0.1
  Gain13 : Gain  Gain=0.016
  Gain14 : Gain  Gain=pi/2
  Gain15 : Gain  Gain=1/2
  Gain16 : Gain  Gain=1/3
  Gain17 : Gain  Gain=-1
  Gain18 : Gain  Gain=-1/2
  Gain19 : Gain  Gain=-1/3
  Gain20 : Gain  Gain=-1/4
  Gain40 : Gain  Gain=-pi*4.75/4
  LCG2 : Math  Operator=square  SignedPower=on  SaturateOnIntegerOverflow=on
  LCG3 : Math  Operator=pow  SignedPower=on  SaturateOnIntegerOverflow=on
  LCG4 : Math  Operator=pow  SignedPower=on  SaturateOnIntegerOverflow=on
  Nr : Gain  Gain=0.02
  Nr' : Gain  Gain=1.2
  Nr|r| : Gain
  Nr|v| : Gain
  Nv : Gain  Gain=0.06
  Nv' : Gain  Gain=2.5
  Nv|r| : Gain
  Nv|v| : Gain
  Product20 : Product
  Product21 : Product  Inputs=*/
  Product22 : Product  Inputs=*/
  Product23 : Product  Inputs=3
  Product24 : Product
  Producto{,3..4,6} (4 alike) : Product
  Producto{1..2,5,7..10} (7 alike) : Product  Inputs=3
  Square{,1..4} (5 alike) : Math  Operator=square  SignedPower=on  SaturateOnIntegerOverflow=on
  Sum{5,19..21,23..24} (6 alike) : Sum  Inputs=|++
  Sum2 : Sum  Inputs=-+++
  Sum22 : Sum  Inputs=|+-
  Sum9 : Sum  Inputs=|+-
  T4 : Math  Operator=pow  SignedPower=on  SaturateOnIntegerOverflow=on
  Terminator : Terminator
  Xu' : Gain  Gain=-0.075
  Yr : Gain  Gain=3
  Yr' : Gain  Gain=0.2
  Yr|r| : Gain
  Yr|v| : Gain
  Yv : Gain  Gain=0.5
  Yv' : Gain  Gain=0.9
  Yv|r| : Gain
  Yv|v| : Gain
  cte : Constant  Value=1.1
  cte1 : Constant  Value=4
  cte2 : Constant  Value=3
  rho*T : Product
  sqrt(u2+v2) : Sqrt  SaturateOnIntegerOverflow=on
  "Hydrodynamic Coefficients " : Outport  VectorParamsAs1DForOutWhenUnconnected=off
  wires:
  m/1 -> Xu'/1
  Nv'/1 -> Bus Creator/4  "N_v_dot"
  Xu'/1 -> Bus Creator/1  "X_u_dot"
  Square/1 -> Gain13/1
  Gain14/1 -> Product23/1
  Product24/1 -> Gain14/1
  Sum9/1 -> (L-LCG)3/1, (L-LCG)4/1, (L-LCG)2/1
  Square4/1 -> Producto2/3
  sqrt(u2+v2)/1 -> Producto2/2, Producto1/2
  Product20/1 -> Product23/2
  Gain13/1 -> Sum2/4
  B_hull/1 -> Producto5/2, Product22/1  "B_hull"
  Square2/1 -> Sum5/2
  Sum20/1 -> Nr'/1
  Gain12/1 -> Sum2/1
  Sum21/1 -> Gain16/1
  LCG4/1 -> Sum24/2
  Sum24/1 -> Producto10/1
  (L-LCG)4/1 -> Sum24/1
  Sum2/1 -> Product23/3
  Producto10/1 -> Gain20/1
  (L-LCG)3/1 -> Sum21/1, Sum23/1
  Producto6/1 -> Sum20/1
  Gain19/1 -> Yr|r|/1, Nr|v|/1, Nv|r|/1
  Gain16/1 -> Producto6/2
  Sum22/1 -> Producto8/2
  Producto3/1 -> Yv'/1
  Gain10/1 -> Product20/1
  cte1/1 -> LCG4/2, T4/2, (L-LCG)4/2
  cte2/1 -> (L-LCG)3/2, LCG3/2
  Product23/1 -> Yv/1
  cte/1 -> Sum2/2
  Producto8/1 -> Gain18/1
  Sum23/1 -> Producto9/1
  Gain20/1 -> Nr|r|/1
  Gain18/1 -> Nv|v|/1, Yr|v|/1, Yv|r|/1
  Yr'/1 -> Bus Creator/3  "Y_r_dot"
  Producto7/1 -> Gain17/1
  Producto9/1 -> Gain19/1
  Gain11/1 -> Sum2/3
  Square1/1 -> Producto/2
  Producto2/1 -> Nr/1
  LCG3/1 -> Sum21/2, Sum23/2
  T4/1 -> Producto5/3
  Gain40/1 -> Sum20/2
  Producto4/1 -> Yr'/1, Nv'/1
  Sum19/1 -> Gain15/1
  Square3/1 -> Sum5/1
  Sum5/1 -> sqrt(u2+v2)/1
  rho/1 -> Producto/1, Gain10/1, Producto5/1, rho*T/1  "rho"
  Abs v1/1 -> Product20/2
  Product21/1 -> Gain11/1
  Gain17/1 -> Yv|v|/1
  (L-LCG)2/1 -> Sum19/1, Sum22/1
  Producto1/1 -> Nv/1, Yr/1
  Product22/1 -> Square/1, Gain12/1
  LCG2/1 -> Sum19/2, Sum22/2
  LCG/1 -> Sum9/2, LCG2/1, LCG3/1, LCG4/1  "LCG"
  Producto/1 -> -pi*rho*T^2/1
  -pi*rho*T^2/1 -> Producto4/1, Producto3/2, Producto2/1, Producto1/1, Producto6/1
  Producto5/1 -> Gain40/1
  Gain15/1 -> Producto4/2
  rho*T/1 -> Producto9/2, Producto10/2, Producto7/3, Producto8/3
  T/1 -> Product21/2, rho*T/2, T4/1, Square1/1, Product22/2, Product24/2  "T"
  L/1 -> Producto7/1, Square4/1, Producto1/3, Producto3/1, Product21/1, Product24/1, Sum9/1  "L"
  C_d/1 -> Producto7/2, Producto8/1, Producto9/3, Producto10/3  "C_d"
  Nv/1 -> Bus Creator/15  "N_v"
  Yv|v|/1 -> Bus Creator/8  "Y_v|v|"
  Yr|r|/1 -> Bus Creator/12  "Y_r|r|"
  Yv/1 -> Bus Creator/10  "Y_v"
  Nv|v|/1 -> Bus Creator/14  "N_v|v|"
  Yr|v|/1 -> Bus Creator/11  "Y_r|v|"
  Nv|r|/1 -> Bus Creator/16  "N_v|r|"
  Yr/1 -> Bus Creator/13  "Y_r"
  Nr|r|/1 -> Bus Creator/19  "N_r|r|"
  Nr/1 -> Bus Creator/18  "N_r"
  Xu|u|/1 -> Bus Creator/7  "X_u|u|"
  Yv|r|/1 -> Bus Creator/9  "Y_v|r|"
  Nr|v|/1 -> Bus Creator/17  "N_r|v|"
  Xu/1 -> Bus Creator/6  "X_u"
  Bus Creator/1 -> "Hydrodynamic Coefficients "/1
  Nr'/1 -> Bus Creator/5  "N_r_dot"
  Yv'/1 -> Bus Creator/2  "Y_v_dot"
  Demux/1 -> Square3/1  "u"
  V local/1 -> Demux/1
  Demux/2 -> Abs v1/1, Square2/1  "v"
  Demux/3 -> Terminator/1  "r"

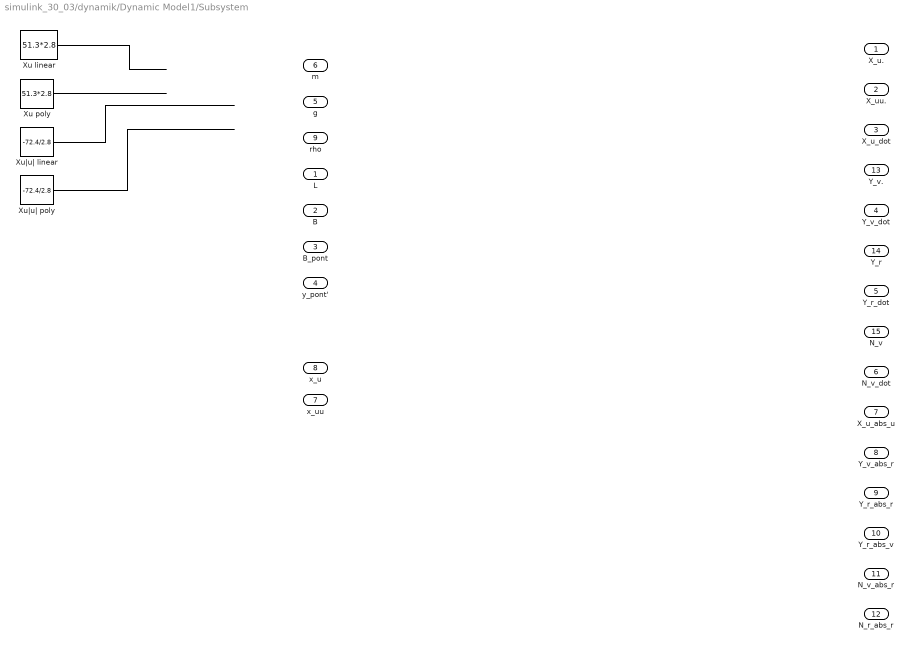
== system simulink_30_03/dynamik/Dynamic Model1/Subsystem ==
  L : Inport
  B : Inport  Port=2
  B_pont : Inport  Port=3
  y_pont' : Inport  Port=4
  g : Inport  Port=5
  m : Inport  Port=6
  x_uu : Inport  Port=7
  x_u : Inport  Port=8
  rho : Inport  Port=9
  Xu linear : Constant  Value=51.3*2.8
  Xu poly : Constant  Value=51.3*2.8
  Xu|u| linear : Constant  Value=-72.4/2.8
  Xu|u| poly : Constant  Value=-72.4/2.8
  X_u. : Outport
  X_uu. : Outport  Port=2
  X_u_dot : Outport  Port=3
  Y_v_dot : Outport  Port=4
  Y_r_dot : Outport  Port=5
  N_v_dot : Outport  Port=6
  X_u_abs_u : Outport  Port=7
  Y_v_abs_r : Outport  Port=8
  Y_r_abs_r : Outport  Port=9
  Y_r_abs_v : Outport  Port=10
  N_v_abs_r : Outport  Port=11
  N_r_abs_r : Outport  Port=12
  Y_v. : Outport  Port=13
  Y_r : Outport  Port=14
  N_v : Outport  Port=15
  wires:
  Xu|u| linear/1 -> ?
  Xu|u| poly/1 -> ?
  Xu poly/1 -> ?
  Xu linear/1 -> ?

== system simulink_30_03/dynamik/Dynamic Model1/Subsystem5 ==
  psi : Inport
  " J(n)" : sharedutil/Create 3x3 Matrix  aMode=aMode
      settings: SourceProductBaseCode=AE,PW,DR,MT,UV,VE
  Constant1 : Constant
  Constant2 : Constant  Value=0
  Gain9 : Gain  Gain=-1
  Selector : Selector  InputPortWidth=3  IndexOptions=Index vector (dialog)  Indices=3  OutputSizes=1
  Trigonometric Function : Trigonometry
  Trigonometric Function1 : Trigonometry  Operator=cos
  J(n) : Outport  VectorParamsAs1DForOutWhenUnconnected=off
  wires:
  Gain9/1 -> " J(n)"/2
  Trigonometric Function1/1 -> " J(n)"/5, " J(n)"/1
  Trigonometric Function/1 -> " J(n)"/4, Gain9/1
  Constant1/1 -> " J(n)"/9
  psi/1 -> Selector/1
  " J(n)"/1 -> J(n)/1
  Constant2/1 -> " J(n)"/8, " J(n)"/7, " J(n)"/6, " J(n)"/3
  Selector/1 -> Trigonometric Function1/1, Trigonometric Function/1

== system simulink_30_03/dynamik/Dynamic Model1/Construct Matrices/M ==
  Hydrodynamic coefficients : Inport
  m1 : Inport  Port=2
  x_g : Inport  Port=3
  y_g : Inport  Port=4
  I_z1 : Inport  Port=5
  Bus Selector : BusSelector  OutputSignals=X_u_dot,Y_r_dot,N_v_dot,Y_v_dot,N_r_dot
  M-matrice : MATLAB Function  TreatAsAtomicUnit=on
  Out_M : Outport
  wires:
  Hydrodynamic coefficients/1 -> Bus Selector/1
  m1/1 -> M-matrice/1(m)
  I_z1/1 -> M-matrice/4(I_z)
  y_g/1 -> M-matrice/3(y_g)
  x_g/1 -> M-matrice/2(x_g)
  M-matrice/1(M_out) -> Out_M/1
  Bus Selector/1 -> M-matrice/5(Xu_dot)  "<X_u_dot>"
  Bus Selector/2 -> M-matrice/7(Yr_dot)  "<Y_r_dot>"
  Bus Selector/4 -> M-matrice/6(Yv_dot)  "<Y_v_dot>"
  Bus Selector/5 -> M-matrice/8(Nr_dot)  "<N_r_dot>"
  Bus Selector/3 -> M-matrice/9(Nv_dot)  "<N_v_dot>"

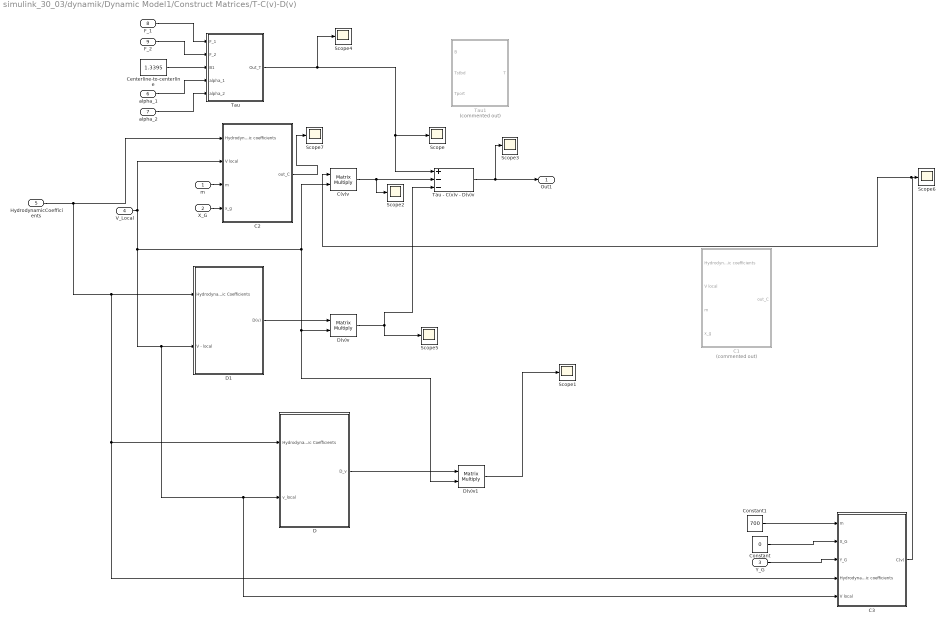
== system simulink_30_03/dynamik/Dynamic Model1/Construct Matrices/T-C(v)-D(v) ==
  m : Inport
  X_G : Inport  Port=2
  Y_G : Inport  Port=3
  V_Local : Inport  Port=4
  HydrodynamicCoefficients : Inport  Port=5
  alpha_1 : Inport  Port=6
  alpha_2 : Inport  Port=7
  F_1 : Inport  Port=8
  F_2 : Inport  Port=9
  C(v)v : Product  Multiplication=Matrix(*)
  C1 : Subsystem  Commented=on
  C2 : Subsystem
  C3 : Subsystem
  Centerline-to-centerline : Constant  Value=1.3395
  Constant : Constant  Value=0
  Constant1 : Constant  Value=700
  D : Subsystem
  D(v)v : Product  Multiplication=Matrix(*)
  D(v)v1 : Product  Multiplication=Matrix(*)
  D1 : Subsystem
  Scope{,1..7} (8 alike) : Scope
  Tau : Subsystem
  Tau - C(v)v - D(v)v : Sum  Inputs=+--
  Tau1 : Subsystem  Commented=on
  Out1 : Outport  VectorParamsAs1DForOutWhenUnconnected=off
  wires:
  V_Local/1 -> C2/2(V local), C3/5(V local), D/2(v_local), D1/2(V - local), D(v)v1/2, D(v)v/2, C(v)v/2
  Tau - C(v)v - D(v)v/1 -> Scope3/1, Out1/1
  HydrodynamicCoefficients/1 -> C2/1(Hydrodynamic coefficients), D/1(Hydrodynamic Coefficients), C3/4(Hydrodynamic coefficients), D1/1(Hydrodynamic Coefficients)
  Centerline-to-centerline/1 -> Tau/3(B1)
  F_2/1 -> Tau/2(F_2)
  F_1/1 -> Tau/1(F_1)
  m/1 -> C2/3(m)
  X_G/1 -> C2/4(x_g)
  Y_G/1 -> C3/3(Y_G)
  C2/1(out_C) -> Scope7/1
  D1/1(D(v)) -> D(v)v/1
  C(v)v/1 -> Scope2/1, Tau - C(v)v - D(v)v/2
  alpha_1/1 -> Tau/4(alpha_1)
  alpha_2/1 -> Tau/5(alpha_2)
  D/1(D_v) -> D(v)v1/1
  D(v)v/1 -> Tau - C(v)v - D(v)v/3, Scope5/1
  D(v)v1/1 -> Scope1/1
  Tau/1(Out_T) -> Scope4/1, Scope/1, Tau - C(v)v - D(v)v/1
  Constant/1 -> C3/2(X_G)
  Constant1/1 -> C3/1(m)
  C3/1(C(v)) -> C(v)v/1, Scope6/1

== system simulink_30_03/dynamik/Dynamic Model1/Construct Matrices/T-C(v)-D(v)/C1 ==
  Hydrodynamic coefficients : Inport
  V local : Inport  Port=2
  m : Inport  Port=3
  x_g : Inport  Port=4
  Demux : Demux  Outputs=19
  Demux1 : Demux  Outputs=3
  MATLAB Function : MATLAB Function  TreatAsAtomicUnit=on
  out_C : Outport
  wires:
  Hydrodynamic coefficients/1 -> Demux/1
  V local/1 -> Demux1/1
  MATLAB Function/1(y) -> out_C/1
  Demux1/1 -> MATLAB Function/2(u)  "u"
  Demux1/2 -> MATLAB Function/1(v)  "v"
  Demux1/3 -> MATLAB Function/3(r)  "r"
  Demux/1 -> MATLAB Function/6(Xu_dot)
  Demux/2 -> MATLAB Function/7(Yv_dot)
  Demux/3 -> MATLAB Function/8(Yr_dot)
  x_g/1 -> MATLAB Function/5(x_g)
  m/1 -> MATLAB Function/4(m)

== system simulink_30_03/dynamik/Dynamic Model1/Construct Matrices/T-C(v)-D(v)/C2 ==
  Hydrodynamic coefficients : Inport
  V local : Inport  Port=2
  m : Inport  Port=3
  x_g : Inport  Port=4
  Demux : Demux  Outputs=19
  Demux1 : Demux  Outputs=3
  MATLAB Function : MATLAB Function  TreatAsAtomicUnit=on
  out_C : Outport
  wires:
  Hydrodynamic coefficients/1 -> Demux/1
  V local/1 -> Demux1/1
  MATLAB Function/1(y) -> out_C/1
  Demux1/1 -> MATLAB Function/2(u)  "u"
  Demux1/2 -> MATLAB Function/1(v)  "v"
  Demux1/3 -> MATLAB Function/3(r)  "r"
  Demux/1 -> MATLAB Function/6(Xu_dot)
  Demux/2 -> MATLAB Function/7(Yv_dot)
  Demux/3 -> MATLAB Function/8(Yr_dot)
  x_g/1 -> MATLAB Function/5(x_g)
  m/1 -> MATLAB Function/4(m)
